simulink model "Controllers_Complete_1"  (R2021a)
settings: Solver=FixedStepAuto  StartTime=vett_t(1)  StopTime=vett_t(end)  FixedStep=0.002  RelTol=1e-3
values from neighbouring files (symbols this model uses):
  sysest_ct = d2c(sysest)    [main.m]
  v_a_max = 10    [main.m]
undefined symbols (not defined in the file or in its folder): HIL, K_comp, Kp, qc_get_step_size, sigbuilder_block, Ti
libraries: simulink_extras x7, quarc_library x4, cstblocks x2
settings Model: Creator=jesuc  LastModifiedBy=arco
settings DataIOCC: SaveFormat=Array  ReturnWorkspaceOutputs=off

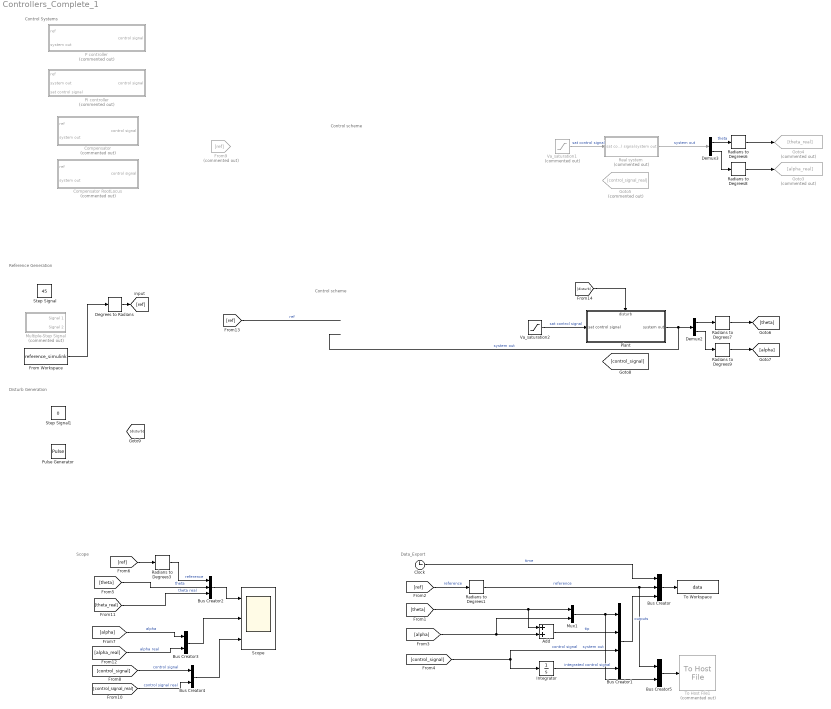
== system Controllers_Complete_1 ==
  note: Control scheme
  note: Control scheme
  note: Scope
  note: Data_Export
  note: Control Systems
  note: Disturb Generation
  note: Reference Generation
  Add : Sum
  Bus Creator : BusCreator  Inputs=3
  Bus Creator1 : BusCreator  Inputs=4
  Bus Creator2 : BusCreator  Inputs=3
  Bus Creator3 : BusCreator  Inputs=2
  Bus Creator4 : BusCreator  Inputs=2
  Bus Creator5 : BusCreator  Inputs=2
  Clock : Clock
  Compensator : Subsystem  Commented=on
  Compensator RootLocus : Subsystem  Commented=on
  Degrees to Radians : simulink_extras/Transformations/Degrees to Radians
  Demux2 : Demux  Outputs=2
  Demux3 : Demux  Outputs=2
  From Workspace : FromWorkspace  VariableName=reference_simulink
  From9 : From  Commented=on  GotoTag=ref
  Goto3 : Goto  Commented=on  GotoTag=alpha_real
  Goto4 : Goto  Commented=on  GotoTag=theta_real
  Goto5 : Goto  Commented=on  GotoTag=control_signal_real
  Integrator : Integrator
  Multiple-Step Signal : Subsystem  Tag=STV Subsys  Commented=on  LoadFcn=sigbuilder_block('load');  StartFcn=sigbuilder_block('start');  StopFcn=sigbuilder_block('stop');  ClipboardFcn=sigbuilder_block('clipboard');  mask(Sigbuilder block){tuvar=[0:10]}
      mask help: Simulink:masks:SigbuilderBlock_MD
      mask init:
      | if ~strcmp(get_param(bdroot(gcbh),'SimulationStatus'),'stopped') tuvar = sigbuilder_block('maskInit'); end
      settings: CopyFcn=sigbuilder_block('copy');  DeleteFcn=sigbuilder_block('delete');  ModelCloseFcn=sigbuilder_block('modelClose');  PreSaveFcn=sigbuilder_block('preSave');  PauseFcn=sigbuilder_block('pause');  ContinueFcn=sigbuilder_block('continue');  NameChangeFcn=sigbuilder_block('namechange');  OpenFcn=sigbuilder_block('open',[6 30 1428 681.75 ]);  CloseFcn=sigbuilder_block('close');
      mask Display: plot(0, 0, 100, 100,[2, 2, 32, 32, 2], [68, 8, 8, 68, 68],[32, 2], [38, 38], [32, 19, 2],[53, 60, 44], [32, 17, 17, 2],[16, 16, 31, 31]);txt = getActiveGroup(gcbh);text(2, 100, txt,'verticalAlignment', 'top');
  Mux1 : Mux  Inputs=2
  P controller : Subsystem  Commented=on
  PI controller : Subsystem  Commented=on
  Plant : Subsystem
      settings: PortSchema="{\"entries\":[{\"content\":{\"sides\":[{\"content\":{\"connectorIds\":[\"In1\"]},\"type\":\"ConnectorPlacement.EquallySpacedRectSide\",\"uuid\":\"cdc36ef1-b9aa-4793-8815-08646de90a91\"},{\"content\":{\"connectorIds\":[\"Out1\"],\"side\":\"RIGHT\"},\"type\":\"ConnectorPlacement.EquallySpacedRectSide\",\"uuid\":\"c826576a-106c-43df-aaf0-aa674a969d04\"},{\"content\":{\"connectorIds\":[\"In2\"],\"side\":\"TOP\"},\"type\":\"ConnectorPlacement.EquallySpacedRectSide\",\"uuid\":\"d2200aa9-f6c9-47e5-a9d0-498ec6850ca3\"}]},\"type\":\"ConnectorPlacement.EquallySpacedConnector\",\"uuid\":\"4474187f-41f3-4590-923f-8ea1970bc9fc\"}],\"packageUris\":[\"http://schema.mathworks.com/mf0/Connector/R2020b\"],\"version\":\"1.0\"}"
  Pulse Generator : DiscretePulseGenerator  PulseType=Time based  Period=10  PulseWidth=5
  Radians to Degrees{1,3,6..9} (6 alike) : simulink_extras/Transformations/Radians to Degrees
  Real system : Subsystem  Commented=on
  Scope : Scope  NumInputPorts=3
  Step Signal : Constant  Value=45
  Step Signal1 : Constant  Value=0
  To Host File1 : quarc_library/Sinks/To Host/To Host File  Commented=on  file_name=Sine tests\Sine_24_in_theta_alpha.mat  variable_name=data  decimation=1  sample_time=-1  file_format=MAT-file v.4  options=No header or footer  append=off  final_file_name=Sine tests\Sine_24_in_theta_alpha.mat  bitrate=2000000
  To Workspace : ToWorkspace  VariableName=data  SampleTime=-1
  Va_saturation1 : Saturate  Commented=on  UpperLimit=v_a_max  LowerLimit=-v_a_max
  Va_saturation2 : Saturate  UpperLimit=v_a_max  LowerLimit=-v_a_max
  wires:
  Va_saturation1/1 -> Real system/1(sat control signal)  "sat control signal"
  Demux3/1 -> Radians to Degrees6/1  "theta"
  ? -> Va_saturation1/1, Goto5/1  "control signal"
  Va_saturation2/1 -> Plant/1(sat control signal)  "sat control signal"
  [disturb] -> Plant/2(disturb)
  ? -> Va_saturation2/1, [control_signal]  "control signal"
  Demux3/2 -> Radians to Degrees8/1
  Radians to Degrees8/1 -> Goto3/1
  Radians to Degrees6/1 -> Goto4/1
  Demux2/2 -> Radians to Degrees9/1
  Radians to Degrees9/1 -> [alpha]
  Plant/1(system out) -> Demux2/1  "system out"
  Radians to Degrees7/1 -> [theta]
  Demux2/1 -> Radians to Degrees7/1
  [alpha] -> Bus Creator3/1  "alpha"
  Integrator/1 -> Bus Creator1/4  "integrated control signal"
  Bus Creator2/1 -> Scope/1
  [control_signal] -> Bus Creator4/1  "control signal"
  [theta] -> Bus Creator2/2  "theta"
  [alpha] -> Add/2, Mux1/2
  [control_signal] -> Integrator/1, Bus Creator1/3  "control signal"
  Bus Creator3/1 -> Scope/2
  Bus Creator4/1 -> Scope/3
  Clock/1 -> Bus Creator/1  "time"
  Add/1 -> Bus Creator1/2  "tip"
  [theta] -> Add/1, Mux1/1
  [theta_real] -> Bus Creator2/3  "theta real"
  Radians to Degrees1/1 -> Bus Creator5/1, Bus Creator/2  "reference"
  Radians to Degrees3/1 -> Bus Creator2/1  "reference"
  [ref] -> Radians to Degrees3/1
  [ref] -> Radians to Degrees1/1  "reference"
  [control_signal_real] -> Bus Creator4/2  "control signal real"
  Bus Creator/1 -> To Workspace/1
  [alpha_real] -> Bus Creator3/2  "alpha real"
  Bus Creator1/1 -> Bus Creator/3  "outputs"
  Bus Creator5/1 -> To Host File1/1
  Mux1/1 -> Bus Creator5/2, Bus Creator1/1  "system out"
  Real system/1(system out) -> Demux3/1  "system out"
  From Workspace/1 -> Degrees to Radians/1
  Degrees to Radians/1 -> [ref]
  [ref] -> ?  "ref"

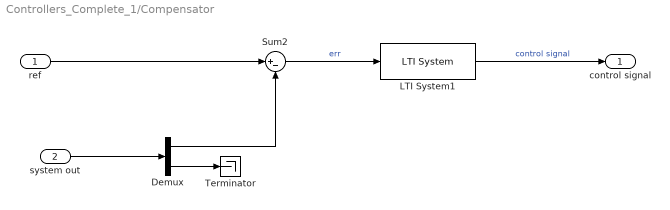
== system Controllers_Complete_1/Compensator ==
  ref : Inport
  system out : Inport  Port=2
  Demux : Demux  Outputs=2
  LTI System1 : cstblocks/LTI System  sys=controller  IC=[]
  Sum2 : Sum  Inputs=|+-
  Terminator : Terminator
  control signal : Outport
  wires:
  LTI System1/1 -> control signal/1  "control signal"
  ref/1 -> Sum2/1
  system out/1 -> Demux/1
  Demux/1 -> Sum2/2
  Sum2/1 -> LTI System1/1  "err"
  Demux/2 -> Terminator/1

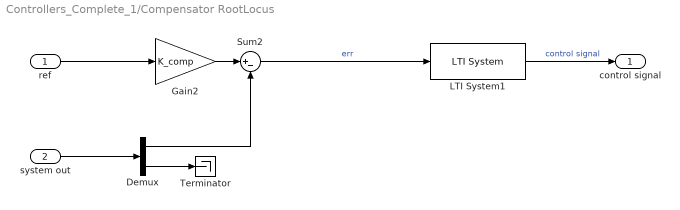
== system Controllers_Complete_1/Compensator RootLocus ==
  ref : Inport
  system out : Inport  Port=2
  Demux : Demux  Outputs=2
  Gain2 : Gain  Gain=K_comp
  LTI System1 : cstblocks/LTI System  sys=controller  IC=[]
  Sum2 : Sum  Inputs=|+-
  Terminator : Terminator
  control signal : Outport
  wires:
  LTI System1/1 -> control signal/1  "control signal"
  system out/1 -> Demux/1
  ref/1 -> Gain2/1
  Demux/1 -> Sum2/2
  Sum2/1 -> LTI System1/1  "err"
  Gain2/1 -> Sum2/1
  Demux/2 -> Terminator/1

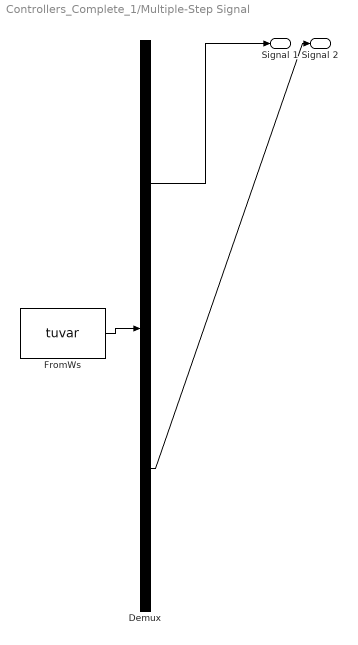
== system Controllers_Complete_1/Multiple-Step Signal ==
  Demux : Demux  Tag=STV Demux  Outputs=2
      settings: DisplayOption=none
  FromWs : FromWorkspace  Tag=STV FromWs  VariableName=tuvar
      SigBuilderData=|
      | common.afterFinalStr = 'Extrapolate'
      | common.sampleTime = 0
      | dataSet.timeRange = [0 10]
      | dataSet.name = 'Group 1'
      | sbobj.Groups.Name = 'Group 1'
      | sbobj.Groups.Signals(1).Name = 'Signal 1'
      | sbobj.Groups.Signals(1).XData = [0 1 1 3 3 7 7 8.5 8.5 10]
      | sbobj.Groups.Signals(1).YData = [0.005 0.005 40 40 -30 -30 0 0 23 23]
      | sbobj.Groups.Signals(2).Name = 'Signal 2'
      | sbobj.Groups.Signals(2).XData = [0 1 1 1.52 10]
      | sbobj.Groups.Signals(2).YData = [0 0 -40 -40 -40]
  Signal 1 : Outport  Tag=STV Outport
  Signal 2 : Outport  Tag=STV Outport  Port=2
  wires:
  Demux/1 -> Signal 1/1
  FromWs/1 -> Demux/1
  Demux/2 -> Signal 2/1

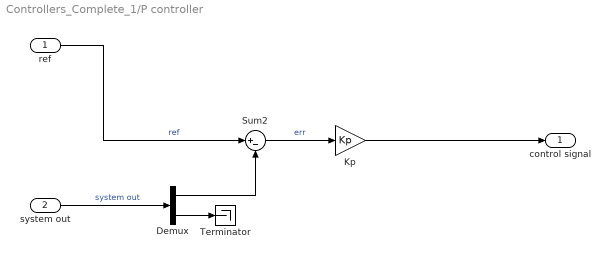
== system Controllers_Complete_1/P controller ==
  ref : Inport
  system out : Inport  Port=2
  Demux : Demux  Outputs=2
  Kp : Gain  Gain=Kp
  Sum2 : Sum  Inputs=|+-
  Terminator : Terminator
  control signal : Outport
  wires:
  Kp/1 -> control signal/1
  Demux/2 -> Terminator/1
  Sum2/1 -> Kp/1  "err"
  Demux/1 -> Sum2/2
  system out/1 -> Demux/1  "system out"
  ref/1 -> Sum2/1  "ref"

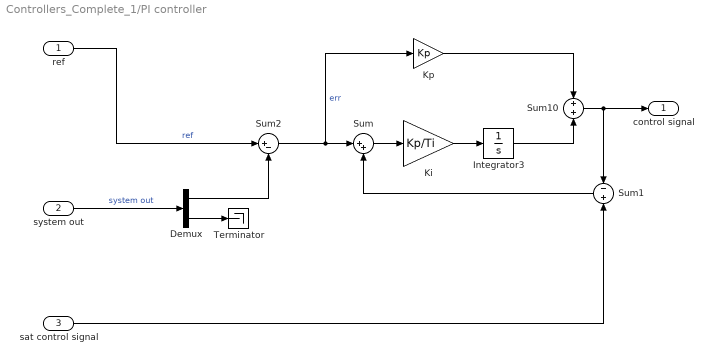
== system Controllers_Complete_1/PI controller ==
  ref : Inport
  system out : Inport  Port=2
  sat control signal : Inport  Port=3
  Demux : Demux  Outputs=2
  Integrator3 : Integrator
  Ki : Gain  Gain=Kp/Ti
  Kp : Gain  Gain=Kp
  Sum : Sum  Inputs=|++
  Sum1 : Sum  Inputs=-+
  Sum10 : Sum
  Sum2 : Sum  Inputs=|+-
  Terminator : Terminator
  control signal : Outport
  wires:
  Ki/1 -> Integrator3/1
  Sum10/1 -> control signal/1, Sum1/1
  Integrator3/1 -> Sum10/2
  Kp/1 -> Sum10/1
  Sum/1 -> Ki/1
  sat control signal/1 -> Sum1/2
  Sum1/1 -> Sum/2
  ref/1 -> Sum2/1  "ref"
  system out/1 -> Demux/1  "system out"
  Demux/2 -> Terminator/1
  Demux/1 -> Sum2/2
  Sum2/1 -> Kp/1, Sum/1  "err"

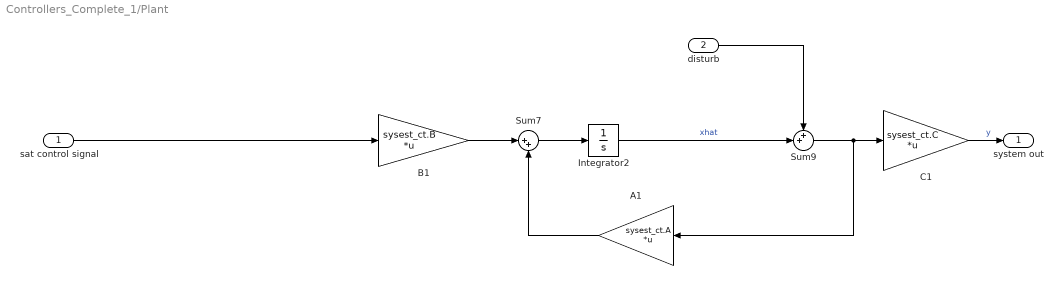
== system Controllers_Complete_1/Plant ==
  sat control signal : Inport
  disturb : Inport  Port=2
  A1 : Gain  Gain=sysest_ct.A  Multiplication=Matrix(K*u)
  B1 : Gain  Gain=sysest_ct.B  Multiplication=Matrix(K*u)
  C1 : Gain  Gain=sysest_ct.C  Multiplication=Matrix(K*u)
  Integrator2 : Integrator
  Sum7 : Sum  Inputs=|++
  Sum9 : Sum  Inputs=++|
  system out : Outport
  wires:
  Sum7/1 -> Integrator2/1
  disturb/1 -> Sum9/1
  B1/1 -> Sum7/1
  Integrator2/1 -> Sum9/2  "xhat"
  C1/1 -> system out/1  "y"
  A1/1 -> Sum7/2
  Sum9/1 -> A1/1, C1/1
  sat control signal/1 -> B1/1

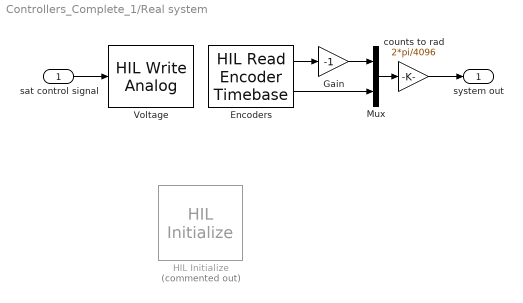
== system Controllers_Complete_1/Real system ==
  sat control signal : Inport
  Encoders : quarc_library/Data Acquisition/Generic/Timebases/HIL Read Encoder Timebase  object_name=HIL-1  clock=0  channels=[0:1]  samples_in_buffer=max(ceil(1/qc_get_step_size), 1)  active=on  vector_output=off  data_type_mode=Inherit via back propagation  data_type=double
  Gain : Gain  Gain=-1
  HIL Initialize : quarc_library/Data Acquisition/Generic/Configuration/HIL Initialize  Priority=-99  Commented=on  object_name=HIL-1  board_type=q2_usb  board_number=0  board_options=d0=digital;d1=digital;led=auto;update_rate=normal;decimation=1  exclusive=off  active=off  hardware_clocks=[0]  clock_modes=[]  initial_clock_frequencies=[]  set_clock_params_at_start=off  set_clock_params_at_switch_in=off  set_clock_frequencies_at_start=off  set_clock_frequencies_at_switch_in=off  analog_input_channels=[0:1]  analog_input_configurations=[]  analog_input_maximums=10  analog_input_minimums=-10  set_analog_input_params_at_start=on  set_analog_input_params_at_switch_in=off  analog_output_channels=[0:1]  analog_output_maximums=10  analog_output_minimums=-10  initial_analog_outputs=[0]  final_analog_outputs=[0]  watchdog_analog_outputs=0  set_analog_output_params_at_start=on  set_analog_output_params_at_switch_in=off  set_analog_outputs_at_start=on  set_analog_outputs_at_switch_in=off  set_analog_outputs_at_terminate=on  set_analog_outputs_at_switch_out=off  set_analog_outputs_on_watchdog=off  digital_input_channels=[]  digital_output_channels=[]  digital_output_configuration=[]  initial_digital_outputs=[1]  final_digital_outputs=[1]  watchdog_digital_outputs=[1]  set_digital_output_params_at_start=off  set_digital_output_params_at_switch_in=off  set_digital_outputs_at_start=on  set_digital_outputs_at_switch_in=off  set_digital_outputs_at_terminate=on  set_digital_outputs_at_switch_out=off  set_digital_outputs_on_watchdog=off  encoder_channels=[0:1]  quadrature=[4]  encoder_filter_frequency=[]  initial_encoder_counts=[0]  set_encoder_params_at_start=on  set_encoder_params_at_switch_in=off  set_encoder_counts_at_start=on  set_encoder_counts_at_switch_in=off  pwm_channels=[]  pwm_modes=[0]  pwm_frequency=1/0.020  pwm_configuration=[]  pwm_alignment=[]  pwm_polarity=[]  pwm_leading_deadband=[]  pwm_trailing_deadband=[]  initial_pwm_outputs=[0]  final_pwm_outputs=[0]  watchdog_pwm_outputs=[0]  set_pwm_params_at_start=on  set_pwm_params_at_switch_in=off  set_pwm_outputs_at_start=on  set_pwm_outputs_at_switch_in=off  set_pwm_outputs_at_terminate=on  set_pwm_outputs_at_switch_out=off  set_pwm_outputs_on_watchdog=off  other_output_channels=[]  initial_other_outputs=[]  final_other_outputs=[]  watchdog_other_outputs=[]  set_other_outputs_at_start=off  set_other_outputs_at_switch_in=off  set_other_outputs_at_terminate=off  set_other_outputs_at_switch_out=off  set_other_outputs_on_watchdog=off
  Mux : Mux  Inputs=2
  Voltage : quarc_library/Data Acquisition/Generic/Immediate I//O/HIL Write Analog  object_name=HIL-1  channels=0  sample_time=-1  active=off  vector_input=off
  counts to rad : Gain  Gain=2*pi/4096
  system out : Outport
  wires:
  sat control signal/1 -> Voltage/1
  Encoders/1 -> Gain/1
  Encoders/2 -> Mux/2
  Mux/1 -> counts to rad/1
  Gain/1 -> Mux/1
  counts to rad/1 -> system out/1
